simulink model "arm"  (R2025b)
settings: Solver=VariableStepAuto  StartTime=0.0  StopTime=10  RelTol=1e-3
values from neighbouring files (symbols this model uses):
  N = length(t)    [generate_cartesian_routine.m]
undefined symbols (not defined in the file or in its folder): X, Y, Z
libraries: sm_lib x16, nesl_utility x10, slpidlib x6
(part 2 of 2)

== matlab function arm/MATLAB Function ==
  data: theta1 output; theta2 output; x input; theta3 output; y input; z input
function [theta1, theta2, theta3] = Inverse_Kinematics(x, y, z)
    % Physical Constants (in meters)
    L0 = 0.05;
    L1 = 0.10; 
    L2 = 0.10;
    % Inverse Kinematics Math (Geometric Approach)
    % Calculate the distance from origin to (x,y)
    r = sqrt(x^2 + y^2);
    h = z - L0;
    D = sqrt(r^2 + h^2);

    %if D > (L1 + L2)
    %    disp('out of reach')
    %end
    % Calculate the terms for acos
    term_beta = (L1^2 + D^2 - L2^2) / (2 * L1 * D);
    term_gamma = (L1^2 + L2^2 - D^2) / (2 * L1 * L2);
   
    % CLAMP: Force the values to stay between -1 and 1
    term_beta = max(min(term_beta, 1), -1);
    term_gamma = max(min(term_gamma, 1), -1);

    % Now calculate the angles safely
    beta = acos(term_beta);
    gamma = acos(term_gamma);
    
    %theta1 (base)
    theta1_rad = atan2(y,x);

    %theta2 (shoulder)
    alpha  = atan2(h,r);
    theta2_rad = alpha + beta;

    %theta3 (elbow)
    theta3_rad = -(pi - gamma);
    
% --- REFERENCE FRAME TRANSLATIONS ---
    
    % theta1 (Base) 
    theta1 = theta1_rad; 
    
    % theta2 (Shoulder):  (0)
    theta2 =  theta2_rad; 
    
    % theta3 (Elbow): Simscape '0' is straight out
    theta3 = theta3_rad;
end
